simulink model "HalfSuspension"  (R2022a)
settings: Solver=ode15s  StartTime=0.0  StopTime=5  MaxStep=1  RelTol=1e-3
values from neighbouring files (symbols this model uses):
  B1 = 1.35    [HalfSuspension_param.m]
  B2 = 1.40    (= 1.4)    [HalfSuspension_param.m]
  C1 = 1500    [HalfSuspension_param.m]
  C2 = 1200    [HalfSuspension_param.m]
  I3 = 418    [HalfSuspension_param.m]
  K1 = 25000    [HalfSuspension_param.m]
  K2 = 20000    [HalfSuspension_param.m]
  KT1 = 200000    [HalfSuspension_param.m]
  KT2 = 180000    [HalfSuspension_param.m]
  M1 = 28    [HalfSuspension_param.m]
  M2 = 28    [HalfSuspension_param.m]
  M3 = 835    [HalfSuspension_param.m]
settings Model: Creator=Orsted  LastModifiedBy=Orsted

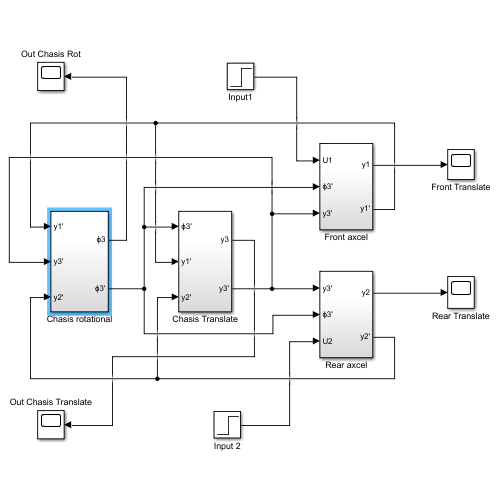
[thumbnail: Simulink's stored preview of the top-level diagram]
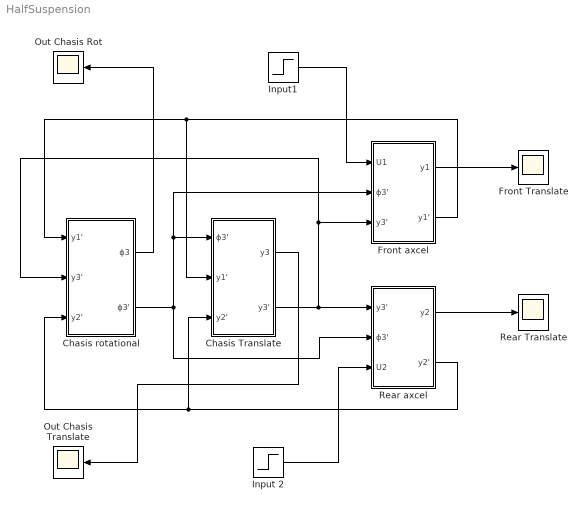
== system HalfSuspension ==
  Chasis Translate : Subsystem
  Chasis rotational : Subsystem
  Front Translate : Scope
  Front axcel : Subsystem
  Input 2 : Step  Time=3  SampleTime=0
  Input1 : Step  SampleTime=0
  Out Chasis Rot : Scope
  Out Chasis Translate : Scope
  Rear Translate : Scope
  Rear axcel : Subsystem
  wires:
  Chasis Translate/2(y3') -> Chasis rotational/2(y3'), Front axcel/3(y3'), Rear axcel/1(y3')
  Chasis rotational/2(ϕ3') -> Front axcel/2(ϕ3'), Chasis Translate/1(ϕ3'), Rear axcel/2(ϕ3')
  Front axcel/2(y1') -> Chasis rotational/1(y1'), Chasis Translate/2(y1')
  Rear axcel/2(y2') -> Chasis rotational/3(y2'), Chasis Translate/3(y2')
  Input 2/1 -> Rear axcel/3(U2)
  Input1/1 -> Front axcel/1(U1)
  Chasis rotational/1(ϕ3) -> Out Chasis Rot/1
  Chasis Translate/1(y3) -> Out Chasis Translate/1
  Front axcel/1(y1) -> Front Translate/1
  Rear axcel/1(y2) -> Rear Translate/1

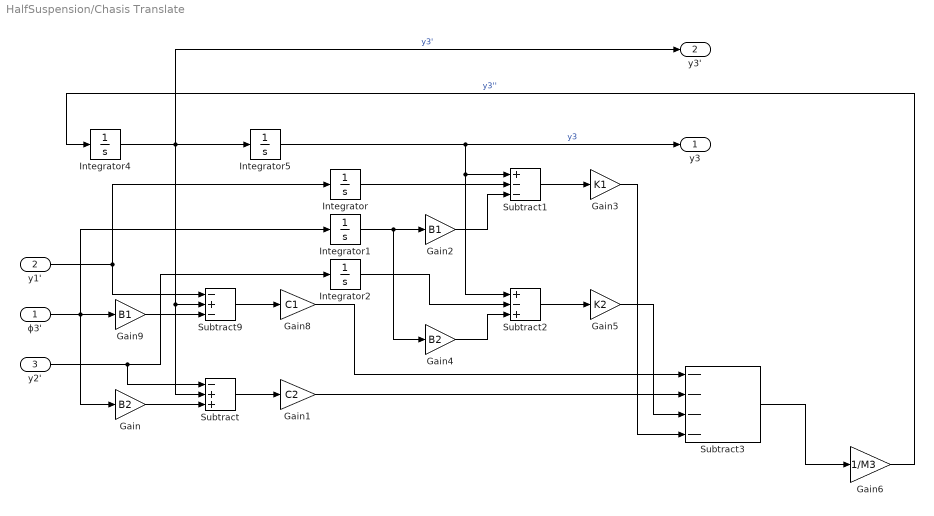
== system HalfSuspension/Chasis Translate ==
  ϕ3' : Inport
  y1' : Inport  Port=2
  y2' : Inport  Port=3
  Gain : Gain  Gain=B2
  Gain1 : Gain  Gain=C2
  Gain2 : Gain  Gain=B1
  Gain3 : Gain  Gain=K1
  Gain4 : Gain  Gain=B2
  Gain5 : Gain  Gain=K2
  Gain6 : Gain  Gain=1/M3
  Gain8 : Gain  Gain=C1
  Gain9 : Gain  Gain=B1
  Integrator{,1..2,4..5} (5 alike) : Integrator
  Subtract : Sum  Inputs=-++
  Subtract1 : Sum  Inputs=+--
  Subtract2 : Sum  Inputs=+-+
  Subtract3 : Sum  Inputs=----
  Subtract9 : Sum  Inputs=-+-
  y3 : Outport
  y3' : Outport  Port=2
  wires:
  Integrator1/1 -> Gain2/1, Gain4/1
  Gain6/1 -> Integrator4/1  "y3''"
  Integrator5/1 -> y3/1, Subtract2/1, Subtract1/1  "y3"
  Gain4/1 -> Subtract2/3
  ϕ3'/1 -> Integrator1/1, Gain/1, Gain9/1
  Subtract1/1 -> Gain3/1
  Gain/1 -> Subtract/3
  Gain9/1 -> Subtract9/3
  y2'/1 -> Integrator2/1, Subtract/1
  Integrator4/1 -> y3'/1, Integrator5/1, Subtract/2, Subtract9/2  "y3'"
  Subtract3/1 -> Gain6/1
  Subtract9/1 -> Gain8/1
  Subtract/1 -> Gain1/1
  Integrator2/1 -> Subtract2/2
  Gain3/1 -> Subtract3/4
  Subtract2/1 -> Gain5/1
  Gain5/1 -> Subtract3/3
  y1'/1 -> Subtract9/1, Integrator/1
  Gain8/1 -> Subtract3/1
  Gain1/1 -> Subtract3/2
  Gain2/1 -> Subtract1/3
  Integrator/1 -> Subtract1/2

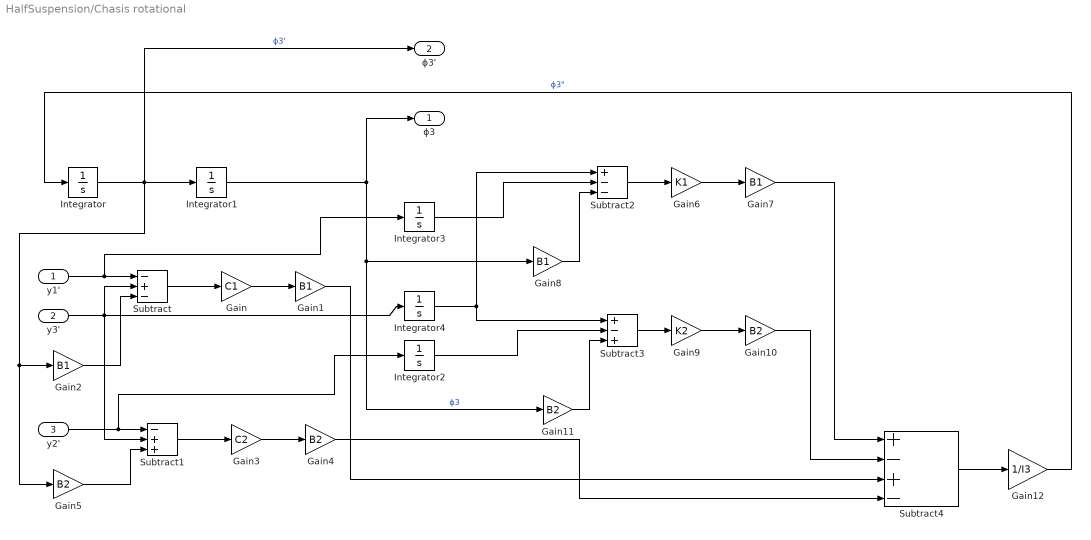
== system HalfSuspension/Chasis rotational ==
  y1' : Inport
  y3' : Inport  Port=2
  y2' : Inport  Port=3
  Gain : Gain  Gain=C1
  Gain{1..2,7..8} (4 alike) : Gain  Gain=B1
  Gain{4..5,10..11} (4 alike) : Gain  Gain=B2
  Gain12 : Gain  Gain=1/I3
  Gain3 : Gain  Gain=C2
  Gain6 : Gain  Gain=K1
  Gain9 : Gain  Gain=K2
  Integrator{,1..4} (5 alike) : Integrator
  Subtract : Sum  Inputs=-+-
  Subtract1 : Sum  Inputs=-++
  Subtract2 : Sum  Inputs=+--
  Subtract3 : Sum  Inputs=+-+
  Subtract4 : Sum  Inputs=+-+-
  ϕ3 : Outport
  ϕ3' : Outport  Port=2
  wires:
  Gain7/1 -> Subtract4/1
  Gain4/1 -> Subtract4/4
  y3'/1 -> Subtract1/2, Integrator4/1, Subtract/2
  Subtract3/1 -> Gain9/1
  Gain5/1 -> Subtract1/3
  Integrator1/1 -> ϕ3/1, Gain11/1, Gain8/1  "ϕ3"
  Subtract/1 -> Gain/1
  Gain2/1 -> Subtract/3
  Integrator3/1 -> Subtract2/2
  y1'/1 -> Integrator3/1, Subtract/1
  y2'/1 -> Integrator2/1, Subtract1/1
  Gain10/1 -> Subtract4/2
  Gain3/1 -> Gain4/1
  Gain6/1 -> Gain7/1
  Integrator2/1 -> Subtract3/2
  Subtract1/1 -> Gain3/1
  Integrator/1 -> ϕ3'/1, Gain2/1, Gain5/1, Integrator1/1  "ϕ3'"
  Gain1/1 -> Subtract4/3
  Subtract4/1 -> Gain12/1
  Gain/1 -> Gain1/1
  Gain9/1 -> Gain10/1
  Gain11/1 -> Subtract3/3
  Gain12/1 -> Integrator/1  "ϕ3\""
  Subtract2/1 -> Gain6/1
  Gain8/1 -> Subtract2/3
  Integrator4/1 -> Subtract3/1, Subtract2/1

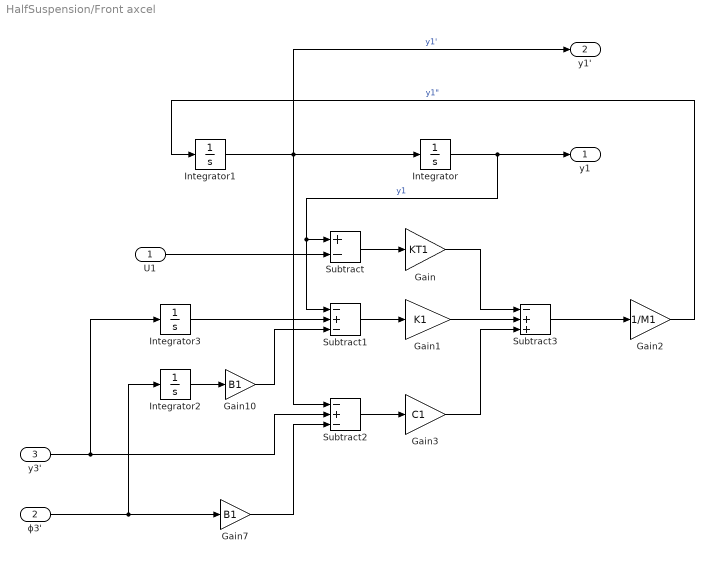
== system HalfSuspension/Front axcel ==
  U1 : Inport
  ϕ3' : Inport  Port=2
  y3' : Inport  Port=3
  Gain : Gain  Gain=KT1
  Gain1 : Gain  Gain=K1
  Gain10 : Gain  Gain=B1
  Gain2 : Gain  Gain=1/M1
  Gain3 : Gain  Gain=C1
  Gain7 : Gain  Gain=B1
  Integrator{,1..3} (4 alike) : Integrator
  Subtract : Sum  Inputs=+-
  Subtract1 : Sum  Inputs=-+-
  Subtract2 : Sum  Inputs=-+-
  Subtract3 : Sum  Inputs=-++
  y1 : Outport
  y1' : Outport  Port=2
  wires:
  Gain1/1 -> Subtract3/2
  Gain/1 -> Subtract3/1
  Gain2/1 -> Integrator1/1  "y1\""
  Integrator/1 -> y1/1, Subtract1/1, Subtract/1  "y1"
  Integrator1/1 -> y1'/1, Subtract2/1, Integrator/1  "y1'"
  Subtract3/1 -> Gain2/1
  ϕ3'/1 -> Integrator2/1, Gain7/1
  Gain3/1 -> Subtract3/3
  U1/1 -> Subtract/2
  Gain7/1 -> Subtract2/3
  Gain10/1 -> Subtract1/3
  Subtract1/1 -> Gain1/1
  Subtract/1 -> Gain/1
  Subtract2/1 -> Gain3/1
  y3'/1 -> Integrator3/1, Subtract2/2
  Integrator2/1 -> Gain10/1
  Integrator3/1 -> Subtract1/2

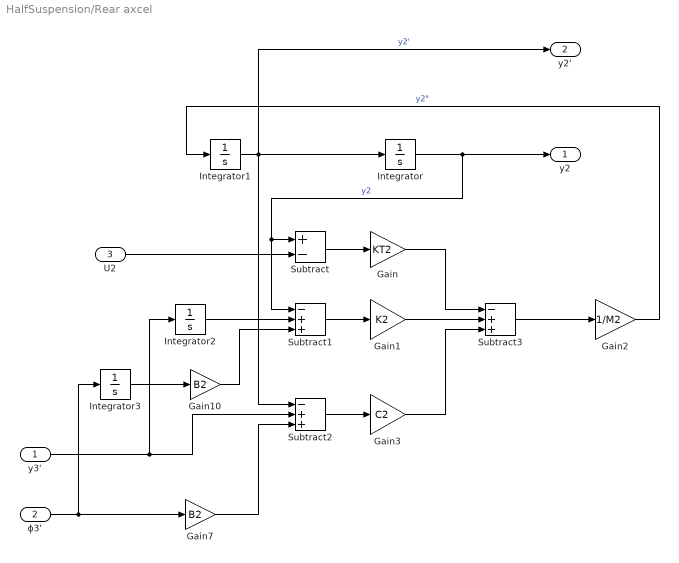
== system HalfSuspension/Rear axcel ==
  y3' : Inport
  ϕ3' : Inport  Port=2
  U2 : Inport  Port=3
  Gain : Gain  Gain=KT2
  Gain1 : Gain  Gain=K2
  Gain10 : Gain  Gain=B2
  Gain2 : Gain  Gain=1/M2
  Gain3 : Gain  Gain=C2
  Gain7 : Gain  Gain=B2
  Integrator{,1..3} (4 alike) : Integrator
  Subtract : Sum  Inputs=+-
  Subtract1 : Sum  Inputs=-++
  Subtract2 : Sum  Inputs=-++
  Subtract3 : Sum  Inputs=-++
  y2 : Outport
  y2' : Outport  Port=2
  wires:
  U2/1 -> Subtract/2
  Subtract2/1 -> Gain3/1
  Gain10/1 -> Subtract1/3
  Subtract1/1 -> Gain1/1
  Gain1/1 -> Subtract3/2
  ϕ3'/1 -> Integrator3/1, Gain7/1
  Subtract3/1 -> Gain2/1
  y3'/1 -> Integrator2/1, Subtract2/2
  Subtract/1 -> Gain/1
  Gain3/1 -> Subtract3/3
  Integrator1/1 -> y2'/1, Subtract2/1, Integrator/1  "y2'"
  Gain7/1 -> Subtract2/3
  Integrator/1 -> y2/1, Subtract1/1, Subtract/1  "y2"
  Gain/1 -> Subtract3/1
  Gain2/1 -> Integrator1/1  "y2\""
  Integrator2/1 -> Subtract1/2
  Integrator3/1 -> Gain10/1
